simulink model "testsim"  (Simulink 8.4)
settings: Solver=ode45  StartTime=0.0  StopTime=10.0  RelTol=1e-6
values from neighbouring files (symbols this model uses):
  A = [0 1 0 0; a 0 0 0; 0 0 0 0; 0 0 1 0]    [testmodel.m]
  B = [B_tau B_d]    [testmodel.m]
  C = Call    [testmodel.m]
  D = zeros(4,2)    [testmodel.m]
  ki = 1/20    (= 0.05)    [testmodel.m]
  L = 0.41    [testmodel.m]
  x10 = 0    [testmodel.m]
  x20 = 0    [testmodel.m]
  x30 = 0    [testmodel.m]
  x40 = 0    [testmodel.m]
settings Model: Creator=elt11jke  LastModifiedBy=frt090_B
settings DebuggingCC: MultiTaskDSMMsg=warning  MultiTaskCondExecSysMsg=none  FcnCallInpInsideContextMsg=EnableAllAsWarning
settings RTWCC: IncludeERTFirstTime=on
settings GRTTargetCC: CombineOutputUpdateFcns=on  GRTInterface=off

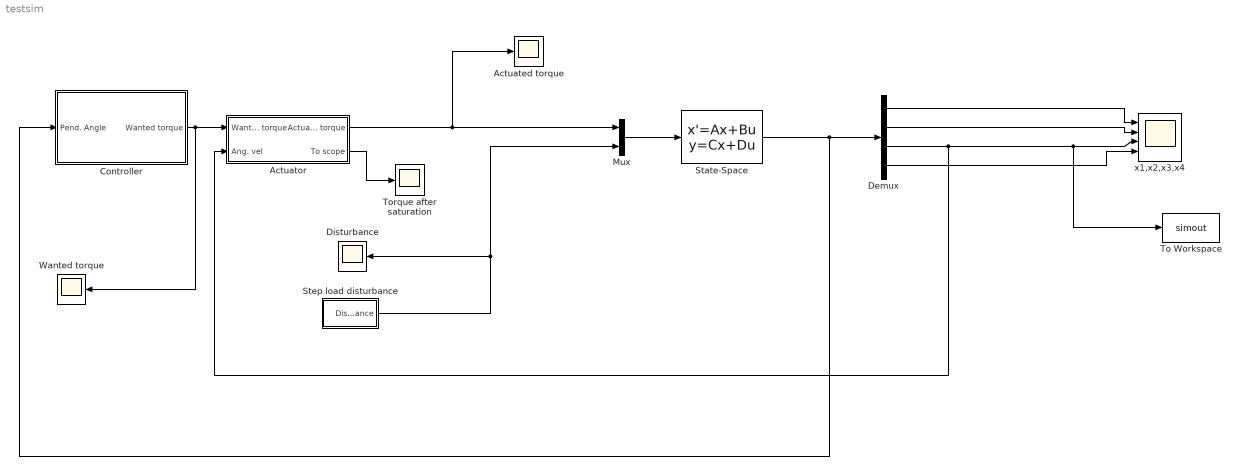
== system testsim ==
  Actuated torque : Scope
      settings: ShowLegends=on  TimeRange=10  YMin=0  YMax=0.00325
  Actuator : Subsystem  TreatAsAtomicUnit=on
  Controller : Subsystem  TreatAsAtomicUnit=on
  Demux : Demux
  Disturbance : Scope
      settings: ShowLegends=on  TimeRange=10  YMin=-0.01  YMax=0.02  SaveName=ScopeData2
  Mux : Mux  Inputs=2
  State-Space : StateSpace  A=A  B=B  C=C  D=D  X0=[x10 x20 x30 x40]
  Step load disturbance : Subsystem
  To Workspace : ToWorkspace  VariableName=simout  SaveFormat=Timeseries  SampleTime=-1
  Torque after saturation : Scope
      settings: ShowLegends=on  TimeRange=10  YMin=0.3648  YMax=0.4032  SaveName=ScopeData4
  Wanted torque : Scope
      settings: ShowLegends=on  TimeRange=10  YMin=-1.355e+07  YMax=-1.3275e+07  SaveName=ScopeData3
  x1,x2,x3,x4 : Scope  NumInputPorts=4
      settings: ShowLegends=on  TimeRange=10  YMin=-6e+38~-6e+39~-20~-5  YMax=2e+38~0~20~5
  wires:
  Demux/1 -> x1,x2,x3,x4/1
  Demux/2 -> x1,x2,x3,x4/2
  Demux/3 -> Actuator/2(Ang. vel), To Workspace/1, x1,x2,x3,x4/3
  Actuator/2(To scope) -> Torque after saturation/1
  Actuator/1(Actuated torque) -> Mux/1, Actuated torque/1
  Step load disturbance/1(Disturbance) -> Mux/2, Disturbance/1
  Controller/1(Wanted torque) -> Actuator/1(Wanted torque), Wanted torque/1
  Mux/1 -> State-Space/1
  State-Space/1 -> Demux/1, Controller/1(Pend. Angle)
  Demux/4 -> x1,x2,x3,x4/4

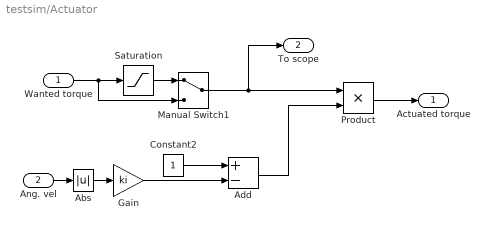
== system testsim/Actuator ==
  Wanted torque : Inport
  Ang. vel : Inport  Port=2
  Abs : Abs
  Add : Sum  Inputs=+-
  Constant2 : Constant
  Gain : Gain  Gain=ki
  Manual Switch1 : ManualSwitch
  Product : Product  RndMeth=Zero
  Saturation : Saturate  UpperLimit=0.384*2  LowerLimit=-0.384*2
  Actuated torque : Outport
  To scope : Outport  Port=2
  wires:
  Wanted torque/1 -> Saturation/1, Manual Switch1/2
  Saturation/1 -> Manual Switch1/1
  Constant2/1 -> Add/1
  Product/1 -> Actuated torque/1
  Add/1 -> Product/2
  Manual Switch1/1 -> Product/1, To scope/1
  Abs/1 -> Gain/1
  Ang. vel/1 -> Abs/1
  Gain/1 -> Add/2

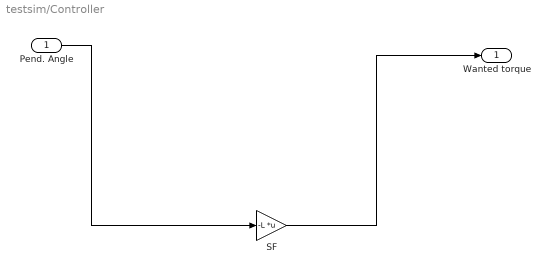
== system testsim/Controller ==
  Pend. Angle : Inport
  SF : Gain  Gain=-L  Multiplication=Matrix(K*u)
  Wanted torque : Outport
  wires:
  SF/1 -> Wanted torque/1
  Pend. Angle/1 -> SF/1

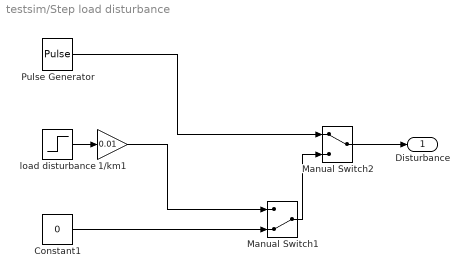
== system testsim/Step load disturbance ==
  1/km1 : Gain  Gain=0.01  SaturateOnIntegerOverflow=on  OutDataTypeStr=Inherit: Same as input  ParamDataTypeStr=Inherit: Same as input
  Constant1 : Constant  Value=0
  Manual Switch1 : ManualSwitch  CurrentSetting=0
  Manual Switch2 : ManualSwitch
  Pulse Generator : DiscretePulseGenerator  PulseType=Time based  Amplitude=0.5  Period=3  PulseWidth=10
  load disturbance : Step  Time=5  After=-0.15  SampleTime=0
  Disturbance : Outport
  wires:
  load disturbance/1 -> 1/km1/1
  Constant1/1 -> Manual Switch1/2
  1/km1/1 -> Manual Switch1/1
  Pulse Generator/1 -> Manual Switch2/1
  Manual Switch1/1 -> Manual Switch2/2
  Manual Switch2/1 -> Disturbance/1
